simulink model "W02_G_lowpass"  (R2024b)
settings: Solver=ode4  StartTime=0  StopTime=lp_T  FixedStep=h  RelTol=1e-3
values from neighbouring files (symbols this model uses):
  lp_a1 = 1    [W02_0_setup.m]
  lp_a2 = 0.3    [W02_0_setup.m]
  lp_w1 = 1    [W02_0_setup.m]
  lp_w2 = 100    [W02_0_setup.m]
  Nf = 20    [W02_0_setup.m]    (also in W02_G_lowpass_filter.m = Nf(i))
settings Model: Creator=admin  LastModifiedBy=admin
settings DataIOCC: ReturnWorkspaceOutputs=off

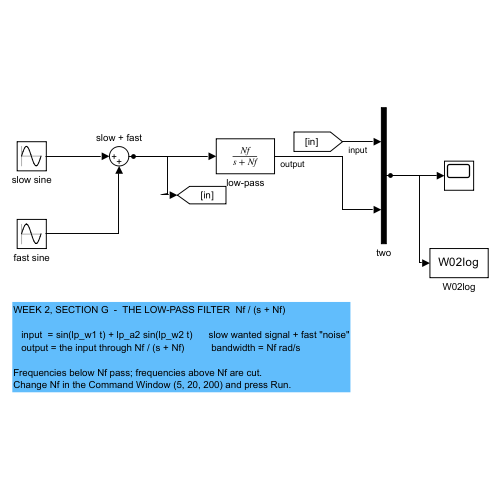
[thumbnail: Simulink's stored preview of the top-level diagram]
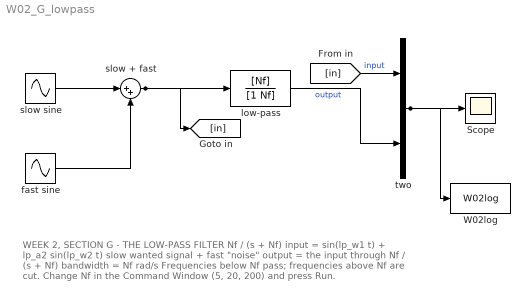
== system W02_G_lowpass ==
  note: WEEK 2, SECTION G  -  THE LOW-PASS FILTER  Nf / (s + Nf)
      |
      |    input  = sin(lp_w1 t) + lp_a2 sin(lp_w2 t)      slow wanted signal + fast "noise"
      |    output = the input through Nf / (s + Nf)          bandwidth = Nf rad/s
      |
      | Frequencies below Nf pass; frequencies above Nf are cut.
      | Change Nf in the Command Window (5, 20, 200) and press Run.
  Scope : Scope
  W02log : ToWorkspace  VariableName=W02log  SaveFormat=Structure With Time  SampleTime=-1
  fast sine : Sin  Amplitude=lp_a2  Frequency=lp_w2  SampleTime=0
  low-pass : TransferFcn  Numerator=[Nf]  Denominator=[1 Nf]
  slow + fast : Sum  Inputs=|++
  slow sine : Sin  Amplitude=lp_a1  Frequency=lp_w1  SampleTime=0
  two : Mux  Inputs=2
  wires:
  slow sine/1 -> slow + fast/1
  fast sine/1 -> slow + fast/2
  slow + fast/1 -> low-pass/1, [in]
  [in] -> two/1  "input"
  low-pass/1 -> two/2  "output"
  two/1 -> Scope/1, W02log/1
